simulink model "Identification_G"  (R2022b)
settings: Solver=ode1  StartTime=0.0  StopTime=14  FixedStep=0.002  RelTol=1e-3  EnableMultiTasking=on
undefined symbols (not defined in the file or in its folder): sigbuilder_block
libraries: quanser_aero x1, simulink_extras x1
settings Model: SimulationMode=external  ExtModeTrigDuration=100000  Creator=MLevis  LastModifiedBy=AERO7
settings SolverCC: AlgebraicLoopSolver=TrustRegion  PositivePriorityOrder=on
settings DataIOCC: SaveFormat=Array  DSMLogging=off  ReturnWorkspaceOutputs=off
settings DebuggingCC: SolverPrmCheckMsg=warning  UnconnectedInputMsg=warning  UnconnectedOutputMsg=warning  UnconnectedLineMsg=warning  SFUnexpectedBacktrackingDiag=warning  SFNoUnconditionalDefaultTransitionDiag=warning  SFExecutionAtInitializationDiag=none  SFMachineParentedDataDiag=warning  ArithmeticOperatorsInVariantConditions=warning
settings ModelReferenceCC: EnableRefExpFcnMdlSchedulingChecks=on  PropagateSignalLabelsOutOfModel=off
settings SFSimCC: SimUseLocalCustomCode=off  CustomCodeUndefinedFunction=UseInterfaceOnly
settings RTWCC: Description=QUARC Win64 Target Using Toolchain  SystemTargetFile=quarc_win64.tlc  TemplateMakefile=quarc_default_tmf  RTWUseLocalCustomCode=off  Toolchain=QUARC win64 | nmake (64-bit Windows)  BuildConfiguration=Faster Runs
settings CodeAppCC: StateflowObjectComments=on
settings STFCustomTargetCC: ConcurrentExecutionCompliant=on  GRTInterface=on  UseToolchainInfoCompliant=on  SystemTargetFile=quarc_win64.tlc
settings GRTTargetCC: TargetLangStandard=C89/C90 (ANSI)  ParMdlRefBuildCompliant=off  CompOptLevelCompliant=off  CombineOutputUpdateFcns=off  MatFileLogging=off  CPPClassGenCompliant=off  GRTInterface=on  ExtMode=on  ExtModeMexFile=quarc_comm
settings ConfigComp: CovMetricSettings=dw  CovSaveCumulativeToWorkspaceVar=on  CovSaveSingleToWorkspaceVar=on  CovExternalEMLEnable=off  CovSFcnEnable=off

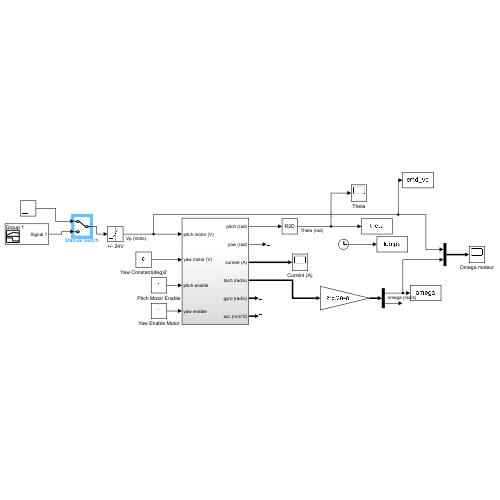
[thumbnail: Simulink's stored preview of the top-level diagram]
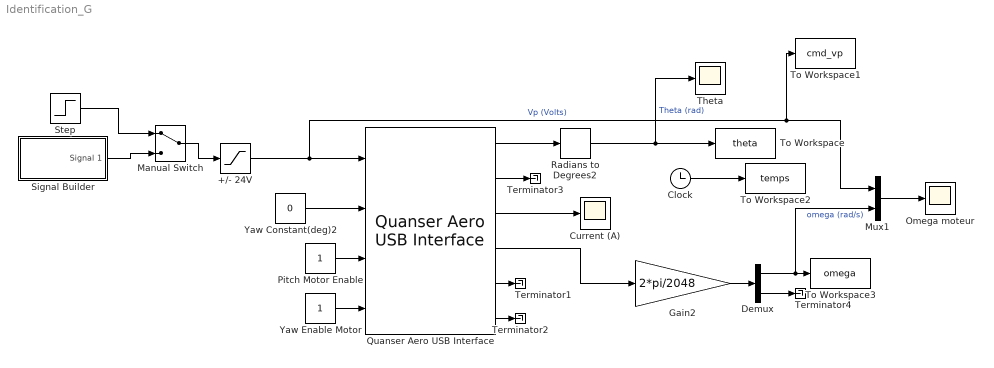
== system Identification_G ==
  +/- 24V : Saturate  UpperLimit=24  LowerLimit=-24
  Clock : Clock
  Current (A) : Scope
  Demux : Demux  Outputs=2
  Gain2 : Gain  Gain=2*pi/2048
  Manual Switch : ManualSwitch
  Mux1 : Mux  Inputs=2
  Omega moteur : Scope
  Pitch Motor Enable : Constant
  Quanser Aero USB Interface : quanser_aero/Quanser Aero USB Interface  SystemSampleTime=-1  VariantActivationTime=update diagram  Latency=0  AutoFrameSizeCalculation=off
  Radians to Degrees2 : simulink_extras/Transformations/Radians to Degrees
  Signal Builder : Subsystem  Tag=STV Subsys  LoadFcn=sigbuilder_block('load');  StartFcn=sigbuilder_block('start');  StopFcn=sigbuilder_block('stop');  ClipboardFcn=sigbuilder_block('clipboard');  mask(Sigbuilder block){tuvar=[0:10]}
      mask help: Simulink:masks:SigbuilderBlock_MD
      mask init:
      | if ~strcmp(get_param(bdroot(gcbh),'SimulationStatus'),'stopped') tuvar = sigbuilder_block('maskInit'); end
      settings: CopyFcn=sigbuilder_block('copy');  DeleteFcn=sigbuilder_block('delete');  ModelCloseFcn=sigbuilder_block('modelClose');  PreSaveFcn=sigbuilder_block('preSave');  PauseFcn=sigbuilder_block('pause');  ContinueFcn=sigbuilder_block('continue');  NameChangeFcn=sigbuilder_block('namechange');  OpenFcn=sigbuilder_block('open',[262.5 120 1092.75 512.25 ]);  CloseFcn=sigbuilder_block('close');
      mask Display: plot(0, 0, 100, 100,[2, 2, 32, 32, 2], [68, 8, 8, 68, 68],[32, 2], [38, 38], [32, 19, 2],[53, 60, 44], [32, 17, 17, 2],[16, 16, 31, 31]);txt = getActiveGroup(gcbh);text(2, 100, txt,'verticalAlignment', 'top');
  Step : Step  After=6  SampleTime=0
  Terminator{1..4} (4 alike) : Terminator
  Theta : Scope
  To Workspace : ToWorkspace  VariableName=theta  SampleTime=-1
      settings: Decimation=10  Save2DSignal=2-D array (concatenate along first dimension)
  To Workspace1 : ToWorkspace  VariableName=cmd_vp  SampleTime=-1
      settings: Decimation=10  Save2DSignal=2-D array (concatenate along first dimension)
  To Workspace2 : ToWorkspace  VariableName=temps  SampleTime=-1
      settings: Decimation=10  Save2DSignal=2-D array (concatenate along first dimension)
  To Workspace3 : ToWorkspace  VariableName=omega  SampleTime=-1
      settings: Decimation=10  Save2DSignal=2-D array (concatenate along first dimension)
  Yaw Constant(deg)2 : Constant  Value=0
  Yaw Enable Motor : Constant
  wires:
  Pitch Motor Enable/1 -> Quanser Aero USB Interface/3
  Yaw Enable Motor/1 -> Quanser Aero USB Interface/4
  Quanser Aero USB Interface/3 -> Current (A)/1
  Quanser Aero USB Interface/1 -> Radians to Degrees2/1
  Quanser Aero USB Interface/4 -> Gain2/1
  Quanser Aero USB Interface/5 -> Terminator1/1
  Quanser Aero USB Interface/6 -> Terminator2/1
  Yaw Constant(deg)2/1 -> Quanser Aero USB Interface/2
  Radians to Degrees2/1 -> Theta/1, To Workspace/1  "Theta (rad)"
  Quanser Aero USB Interface/2 -> Terminator3/1
  Clock/1 -> To Workspace2/1
  Gain2/1 -> Demux/1
  Demux/1 -> Mux1/2, To Workspace3/1  "omega (rad/s)"
  Demux/2 -> Terminator4/1
  Manual Switch/1 -> +/- 24V/1
  Step/1 -> Manual Switch/1
  Mux1/1 -> Omega moteur/1
  +/- 24V/1 -> To Workspace1/1, Mux1/1, Quanser Aero USB Interface/1  "Vp (Volts)"
  Signal Builder/1(Signal 1) -> Manual Switch/2

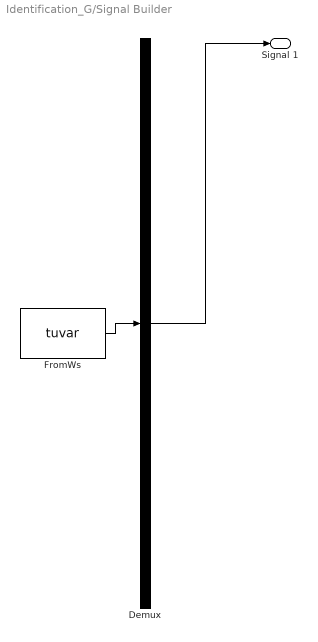
== system Identification_G/Signal Builder ==
  Demux : Demux  Tag=STV Demux  Outputs=1
      settings: DisplayOption=none
  FromWs : FromWorkspace  Tag=STV FromWs  VariableName=tuvar
      SigBuilderData=|
      | common.afterFinalStr = 'Extrapolate'
      | common.sampleTime = 0
      | dataSet.timeRange = [0 14]
      | dataSet.name = 'Group 1'
      | sbobj.Groups.Name = 'Group 1'
      | sbobj.Groups.Signals.Name = 'Signal 1'
      | sbobj.Groups.Signals.XData = [0 1 1 4 4 7 7 10 10 14]
      | sbobj.Groups.Signals.YData = [0 0 2.5 2.5 4.95 5 7.5 7.5 10 10]
      | sbobj.Groups.TimeRange = [0 14]
  Signal 1 : Outport  Tag=STV Outport  VectorParamsAs1DForOutWhenUnconnected=off
  wires:
  Demux/1 -> Signal 1/1
  FromWs/1 -> Demux/1
